simulink model "Vaxelriktare_Transducers"  (R2020b)
settings: Solver=VariableStepAuto  StartTime=0.0  StopTime=0.01  RelTol=1e-3
libraries: fl_lib x80, nesl_utility x32, ee_lib x3, SignalEditorBlockLib x1
(part 1 of 2)
settings Model: Creator=jenel  LastModifiedBy=jenel

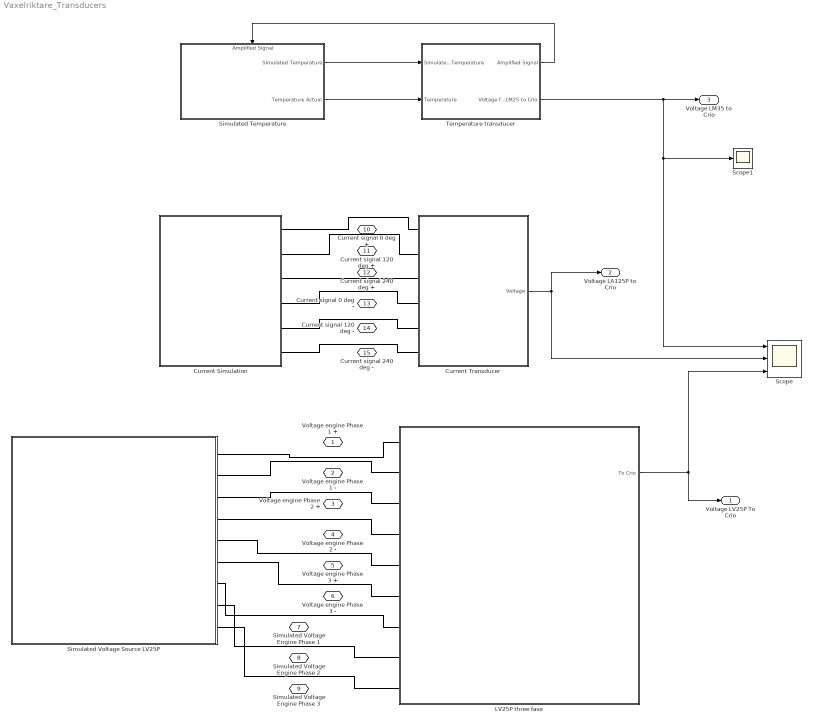
== system Vaxelriktare_Transducers ==
  Current Simulation : Subsystem
  Current Transducer : Subsystem
  LV25P three fase : Subsystem
  Scope : Scope  NumInputPorts=3
  Scope1 : Scope
  Simulated Temperature : Subsystem
      settings: PortSchema="{\"entries\":[{\"content\":{\"sides\":[{\"content\":{\"connectorIds\":[]},\"type\":\"ConnectorPlacement.EquallySpacedRectSide\",\"uuid\":\"52a7c08e-3c3e-468d-9a48-5db7e5268e65\"},{\"content\":{\"connectorIds\":[\"Out1\",\"Out2\"],\"side\":\"RIGHT\"},\"type\":\"ConnectorPlacement.EquallySpacedRectSide\",\"uuid\":\"cc00ce28-dfa9-4e8d-849b-21a8aa2e88a1\"},{\"content\":{\"connectorIds\":[\"In1\"],\"side\":\"TOP\"},\"type\":\"ConnectorPlacement.EquallySpacedRectSide\",\"uuid\":\"9c60ff72-e0ca-4689-b1b7-e246b8e0f47f\"},{\"content\":{\"connectorIds\":[],\"side\":\"HIDDEN\"},\"type\":\"ConnectorPlacement.EquallySpacedRectSide\",\"uuid\":\"4ba62725-7915-4645-8693-141a674fd740\"}]},\"type\":\"ConnectorPlacement.EquallySpacedConnector\",\"uuid\":\"cdec1a03-c0d5-4421-a983-90e94124080d\"}],\"packageUris\":[\"http://schema.mathworks.com/mf0/Connector/R2020b\"],\"version\":\"1.0\"}"
  Simulated Voltage Source LV25P : Subsystem
  Temperature transducer : Subsystem
  Voltage engine Phase 1 + : PMIOPort  Side=Right
  Voltage engine Phase 1 - : PMIOPort  Port=2  Side=Right
  Voltage engine Phase 2 + : PMIOPort  Port=3  Side=Right
  Voltage engine Phase 2 - : PMIOPort  Port=4  Side=Right
  Voltage engine Phase 3 + : PMIOPort  Port=5  Side=Right
  Voltage engine Phase 3 - : PMIOPort  Port=6  Side=Right
  Simulated Voltage Engine Phase 1 : PMIOPort  Port=7  Side=Right
  Simulated Voltage Engine Phase 2 : PMIOPort  Port=8  Side=Right
  Simulated Voltage Engine Phase 3 : PMIOPort  Port=9  Side=Right
  Current signal 0 deg + : PMIOPort  Port=10  Side=Right
  Current signal 120 deg + : PMIOPort  Port=11  Side=Right
  Current signal 240 deg + : PMIOPort  Port=12  Side=Right
  Current signal 0 deg - : PMIOPort  Port=13  Side=Right
  Current signal 120 deg - : PMIOPort  Port=14  Side=Right
  Current signal 240 deg - : PMIOPort  Port=15  Side=Right
  Voltage LV25P To Crio : Outport
  Voltage LA125P to Crio : Outport  Port=2
  Voltage LM35 to Crio : Outport  Port=3
  wires:
  LV25P three fase/1(To Crio) -> Voltage LV25P To Crio/1, Scope/3
  Current Transducer/1(Voltage) -> Scope/2, Voltage LA125P to Crio/1
  Simulated Temperature/1(Simulated Temperature) -> Temperature transducer/1(Simulated Temperature)
  Simulated Temperature/2(Temperature Actual) -> Temperature transducer/2(Temperature)
  Temperature transducer/1(Amplified Signal) -> Simulated Temperature/1(Amplified Signal)
  Temperature transducer/2(Voltage from LM25 to Crio) -> Voltage LM35 to Crio/1, Scope1/1, Scope/1
  connections:
  Simulated Voltage Source LV25P/RConn2 -- LV25P three fase/LConn2
  Simulated Voltage Source LV25P/RConn5 -- LV25P three fase/LConn5
  Simulated Voltage Source LV25P/RConn4 -- LV25P three fase/LConn4
  LV25P three fase/LConn6 -- Simulated Voltage Source LV25P/RConn6
  LV25P three fase/LConn7 -- Simulated Voltage Source LV25P/RConn7
  Simulated Voltage Source LV25P/RConn8 -- LV25P three fase/LConn8
  LV25P three fase/LConn3 -- Simulated Voltage Source LV25P/RConn3
  Simulated Voltage Source LV25P/RConn9 -- LV25P three fase/LConn9
  LV25P three fase/LConn1 -- Simulated Voltage Source LV25P/RConn1
  Current Simulation/LConn3 -- Current Transducer/LConn3
  Current Simulation/LConn2 -- Current Transducer/LConn2
  Current Simulation/LConn1 -- Current Transducer/LConn1
  Current Simulation/LConn6 -- Current Transducer/LConn6
  Current Simulation/LConn5 -- Current Transducer/LConn5
  Current Simulation/LConn4 -- Current Transducer/LConn4

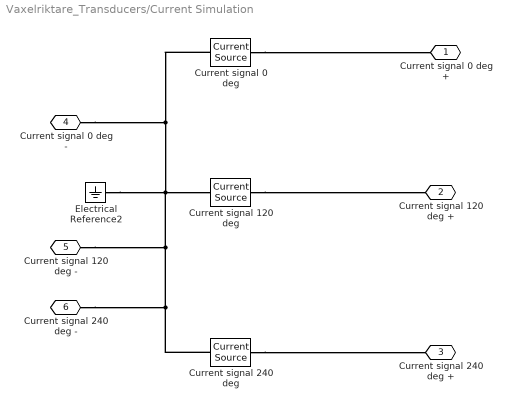
== system Vaxelriktare_Transducers/Current Simulation ==
  Current signal 0 deg : ee_lib/Sources/Current Source  dc_current=0 A  ac_current=200 mA  ac_shift=0 deg  ac_frequency=1000 Hz  noise_mode=0  PSD=0 A^2/Hz  repeatability=1  auto_seed=1274213173  user_seed=0  sample_time=1e-3 s  i_specify=off  i_priority=None  i=0 A  i_nominal_specify=off  i_nominal_unit=A  i_nominal_value=1  v_specify=off  v_priority=None  v=0 V  v_nominal_specify=off  v_nominal_unit=V  v_nominal_value=1
      settings: SourceProductBaseCode=PS
  Current signal 120 deg : ee_lib/Sources/Current Source  dc_current=0 A  ac_current=200 mA  ac_shift=120 deg  ac_frequency=1000 Hz  noise_mode=0  PSD=0 A^2/Hz  repeatability=1  auto_seed=1369142382  user_seed=0  sample_time=1e-3 s  i_specify=off  i_priority=None  i=0 A  i_nominal_specify=off  i_nominal_unit=A  i_nominal_value=1  v_specify=off  v_priority=None  v=0 V  v_nominal_specify=off  v_nominal_unit=V  v_nominal_value=1
      settings: SourceProductBaseCode=PS
  Current signal 240 deg : ee_lib/Sources/Current Source  dc_current=0 A  ac_current=200 mA  ac_shift=240 deg  ac_frequency=1000 Hz  noise_mode=0  PSD=0 A^2/Hz  repeatability=1  auto_seed=1821782361  user_seed=0  sample_time=1e-3 s  i_specify=off  i_priority=None  i=0 A  i_nominal_specify=off  i_nominal_unit=A  i_nominal_value=1  v_specify=off  v_priority=None  v=0 V  v_nominal_specify=off  v_nominal_unit=V  v_nominal_value=1
      settings: SourceProductBaseCode=PS
  Electrical Reference2 : fl_lib/Electrical/Electrical Elements/Electrical Reference
  Current signal 0 deg + : PMIOPort  Side=Left
  Current signal 120 deg + : PMIOPort  Port=2  Side=Left
  Current signal 240 deg + : PMIOPort  Port=3  Side=Left
  Current signal 0 deg - : PMIOPort  Port=4  Side=Left
  Current signal 120 deg - : PMIOPort  Port=5  Side=Left
  Current signal 240 deg - : PMIOPort  Port=6  Side=Left
  connections:
  Electrical Reference2/LConn1 -- Current signal 0 deg/RConn1 -- Current signal 0 deg -/RConn1 -- Current signal 240 deg/RConn1 -- Current signal 240 deg -/RConn1 -- Current signal 120 deg -/RConn1 -- Current signal 120 deg/RConn1
  Current signal 240 deg/LConn1 -- Current signal 240 deg +/RConn1
  Current signal 0 deg/LConn1 -- Current signal 0 deg +/RConn1
  Current signal 120 deg/LConn1 -- Current signal 120 deg +/RConn1

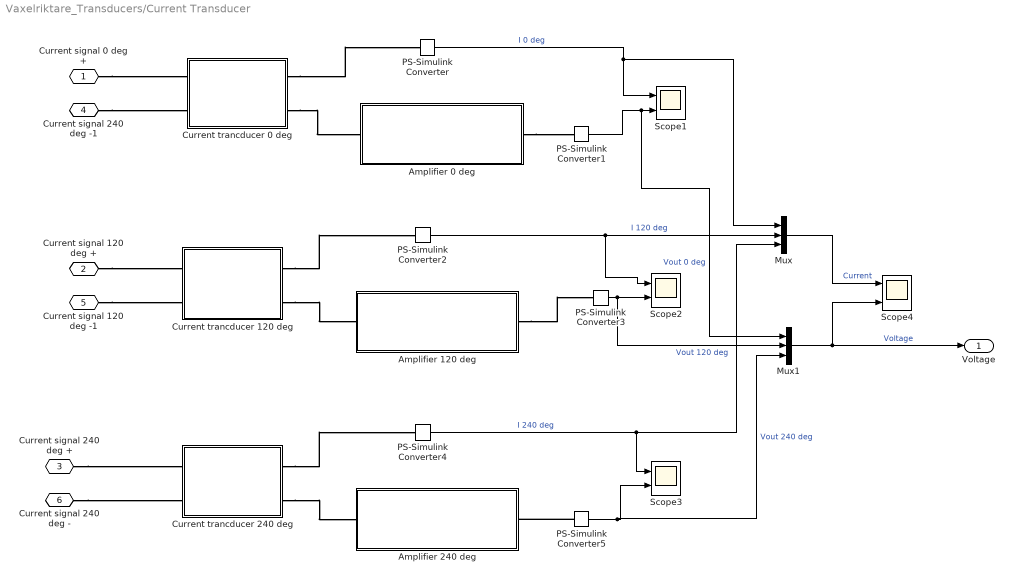
== system Vaxelriktare_Transducers/Current Transducer ==
  Amplifier 0 deg : Subsystem
  Amplifier 120 deg : Subsystem
  Amplifier 240 deg : Subsystem
  Current trancducer 0 deg : Subsystem
  Current trancducer 120 deg : Subsystem
  Current trancducer 240 deg : Subsystem
  Mux : Mux  Inputs=3
  Mux1 : Mux  Inputs=3
  PS-Simulink Converter{,1..5} (6 alike) : nesl_utility/PS-Simulink Converter  PhysicalDomain=network_engine_domain  SubClassName=ps_output  LeftPortType=input  RightPortType=output  PseudoPeriodic=off  Frequencies=[]  Unit=inherit  AffineConversion=off
  Scope{1..4} (4 alike) : Scope  NumInputPorts=2
  Current signal 0 deg + : PMIOPort  Side=Left
  Current signal 120 deg + : PMIOPort  Port=2  Side=Left
  Current signal 240 deg + : PMIOPort  Port=3  Side=Left
  Current signal 240 deg -1 : PMIOPort  Port=4  Side=Left
  Current signal 120 deg -1 : PMIOPort  Port=5  Side=Left
  Current signal 240 deg - : PMIOPort  Port=6  Side=Left
  Voltage : Outport
  wires:
  PS-Simulink Converter1/1 -> Mux1/1, Scope1/2  "Vout 0 deg"
  PS-Simulink Converter5/1 -> Mux1/3, Scope3/2  "Vout 240 deg"
  PS-Simulink Converter3/1 -> Mux1/2, Scope2/2  "Vout 120 deg"
  PS-Simulink Converter/1 -> Mux/1, Scope1/1  "I 0 deg"
  PS-Simulink Converter2/1 -> Scope2/1, Mux/2  "I 120 deg"
  PS-Simulink Converter4/1 -> Mux/3, Scope3/1  "I 240 deg"
  Mux1/1 -> Voltage/1, Scope4/2  "Voltage"
  Mux/1 -> Scope4/1  "Current"
  connections:
  Amplifier 120 deg/RConn1 -- PS-Simulink Converter3/LConn1
  Current trancducer 120 deg/RConn2 -- Amplifier 120 deg/LConn1
  Current trancducer 0 deg/RConn2 -- Amplifier 0 deg/LConn1
  Current trancducer 120 deg/RConn1 -- PS-Simulink Converter2/LConn1
  Current trancducer 0 deg/RConn1 -- PS-Simulink Converter/LConn1
  Current trancducer 240 deg/RConn2 -- Amplifier 240 deg/LConn1
  PS-Simulink Converter5/LConn1 -- Amplifier 240 deg/RConn1
  Amplifier 0 deg/RConn1 -- PS-Simulink Converter1/LConn1
  Current trancducer 240 deg/RConn1 -- PS-Simulink Converter4/LConn1
  Current signal 0 deg +/RConn1 -- Current trancducer 0 deg/LConn1
  Current signal 120 deg +/RConn1 -- Current trancducer 120 deg/LConn1
  Current signal 240 deg +/RConn1 -- Current trancducer 240 deg/LConn1
  Current signal 240 deg -/RConn1 -- Current trancducer 240 deg/LConn2
  Current signal 120 deg -1/RConn1 -- Current trancducer 120 deg/LConn2
  Current signal 240 deg -1/RConn1 -- Current trancducer 0 deg/LConn2

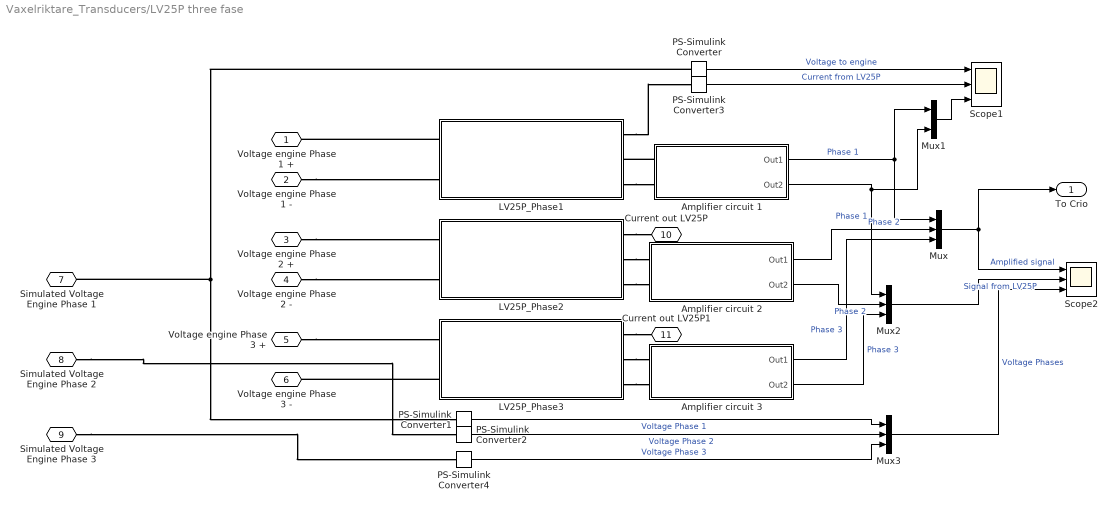
== system Vaxelriktare_Transducers/LV25P three fase ==
  Amplifier circuit 1 : Subsystem
  Amplifier circuit 2 : Subsystem
  Amplifier circuit 3 : Subsystem
  LV25P_Phase1 : Subsystem
  LV25P_Phase2 : Subsystem
  LV25P_Phase3 : Subsystem
  Mux : Mux  Inputs=3
  Mux1 : Mux  Inputs=2
  Mux2 : Mux  Inputs=3
  Mux3 : Mux  Inputs=3
  PS-Simulink Converter{,1..4} (5 alike) : nesl_utility/PS-Simulink Converter  PhysicalDomain=network_engine_domain  SubClassName=ps_output  LeftPortType=input  RightPortType=output  PseudoPeriodic=off  Frequencies=[]  Unit=inherit  AffineConversion=off
  Scope1 : Scope  NumInputPorts=3
  Scope2 : Scope  NumInputPorts=3
  Voltage engine Phase 1 + : PMIOPort  Side=Left
  Voltage engine Phase 1 - : PMIOPort  Port=2  Side=Left
  Voltage engine Phase 2 + : PMIOPort  Port=3  Side=Left
  Voltage engine Phase 2 - : PMIOPort  Port=4  Side=Left
  Voltage engine Phase 3 + : PMIOPort  Port=5  Side=Left
  Voltage engine Phase 3 - : PMIOPort  Port=6  Side=Left
  Simulated Voltage Engine Phase 1 : PMIOPort  Port=7  Side=Left
  Simulated Voltage Engine Phase 2 : PMIOPort  Port=8  Side=Left
  Simulated Voltage Engine Phase 3 : PMIOPort  Port=9  Side=Left
  Current out LV25P : PMIOPort  Port=10  Side=Right
  Current out LV25P1 : PMIOPort  Port=11  Side=Right
  To Crio : Outport
  wires:
  Mux3/1 -> Scope2/3  "Voltage Phases"
  PS-Simulink Converter1/1 -> Mux3/1  "Voltage Phase 1"
  Amplifier circuit 3/1(Out1) -> Mux/3  "Phase 3"
  Mux/1 -> To Crio/1, Scope2/1  "Amplified signal"
  PS-Simulink Converter4/1 -> Mux3/3  "Voltage Phase 3"
  Mux1/1 -> Scope1/3
  Amplifier circuit 1/2(Out2) -> Mux2/1, Mux1/2  "Phase 1"
  Amplifier circuit 2/2(Out2) -> Mux2/2  "Phase 2"
  PS-Simulink Converter2/1 -> Mux3/2  "Voltage Phase 2"
  PS-Simulink Converter/1 -> Scope1/1  "Voltage to engine"
  PS-Simulink Converter3/1 -> Scope1/2  "Current from LV25P"
  Amplifier circuit 2/1(Out1) -> Mux/2  "Phase 2"
  Amplifier circuit 3/2(Out2) -> Mux2/3  "Phase 3"
  Mux2/1 -> Scope2/2  "Signal from LV25P"
  Amplifier circuit 1/1(Out1) -> Mux1/1, Mux/1  "Phase 1"
  connections:
  Amplifier circuit 1/LConn1 -- LV25P_Phase1/RConn2
  Voltage engine Phase 2 -/RConn1 -- LV25P_Phase2/LConn2
  LV25P_Phase3/LConn2 -- Voltage engine Phase 3 -/RConn1
  LV25P_Phase2/RConn2 -- Amplifier circuit 2/LConn1
  PS-Simulink Converter/LConn1 -- PS-Simulink Converter1/LConn1 -- Simulated Voltage Engine Phase 1/RConn1
  LV25P_Phase1/RConn3 -- Amplifier circuit 1/LConn2
  LV25P_Phase2/RConn3 -- Amplifier circuit 2/LConn2
  Voltage engine Phase 3 +/RConn1 -- LV25P_Phase3/LConn1
  Simulated Voltage Engine Phase 3/RConn1 -- PS-Simulink Converter4/LConn1
  LV25P_Phase1/RConn1 -- PS-Simulink Converter3/LConn1
  Simulated Voltage Engine Phase 2/RConn1 -- PS-Simulink Converter2/LConn1
  Voltage engine Phase 2 +/RConn1 -- LV25P_Phase2/LConn1
  Voltage engine Phase 1 -/RConn1 -- LV25P_Phase1/LConn2
  LV25P_Phase1/LConn1 -- Voltage engine Phase 1 +/RConn1
  LV25P_Phase3/RConn2 -- Amplifier circuit 3/LConn1
  LV25P_Phase3/RConn3 -- Amplifier circuit 3/LConn2
  LV25P_Phase2/RConn1 -- Current out LV25P/RConn1
  LV25P_Phase3/RConn1 -- Current out LV25P1/RConn1

== system Vaxelriktare_Transducers/Simulated Temperature ==
  Amplified Signal : Inport
  Calculation temperature : Subsystem
  Mux1 : Mux  Inputs=2
  Temperature Simulation 2-150C : Subsystem
  Simulated Temperature : Outport
  Temperature Actual : Outport  Port=2
  wires:
  Temperature Simulation 2-150C/1(output) -> Temperature Actual/1, Mux1/2  "Temperature Actual"
  Calculation temperature/1(Temperature Measured) -> Mux1/1
  Mux1/1 -> Simulated Temperature/1
  Amplified Signal/1 -> Calculation temperature/1(Amplified Signal)

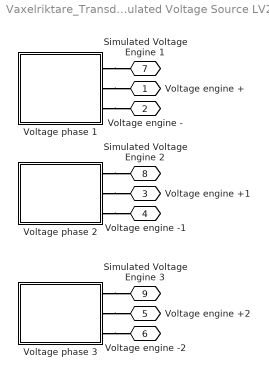
== system Vaxelriktare_Transducers/Simulated Voltage Source LV25P ==
  Voltage phase 1 : Subsystem
  Voltage phase 2 : Subsystem
  Voltage phase 3 : Subsystem
  Voltage engine + : PMIOPort  Side=Right
  Voltage engine - : PMIOPort  Port=2  Side=Right
  Voltage engine +1 : PMIOPort  Port=3  Side=Right
  Voltage engine -1 : PMIOPort  Port=4  Side=Right
  Voltage engine +2 : PMIOPort  Port=5  Side=Right
  Voltage engine -2 : PMIOPort  Port=6  Side=Right
  Simulated Voltage Engine 1 : PMIOPort  Port=7  Side=Right
  Simulated Voltage Engine 2 : PMIOPort  Port=8  Side=Right
  Simulated Voltage Engine 3 : PMIOPort  Port=9  Side=Right
  connections:
  Voltage phase 1/RConn3 -- Voltage engine -/RConn1
  Voltage phase 2/RConn3 -- Voltage engine -1/RConn1
  Voltage phase 2/RConn1 -- Simulated Voltage Engine 2/RConn1
  Voltage phase 3/RConn1 -- Simulated Voltage Engine 3/RConn1
  Voltage phase 1/RConn1 -- Simulated Voltage Engine 1/RConn1
  Voltage phase 1/RConn2 -- Voltage engine +/RConn1
  Voltage phase 3/RConn3 -- Voltage engine -2/RConn1
  Voltage phase 3/RConn2 -- Voltage engine +2/RConn1
  Voltage phase 2/RConn2 -- Voltage engine +1/RConn1

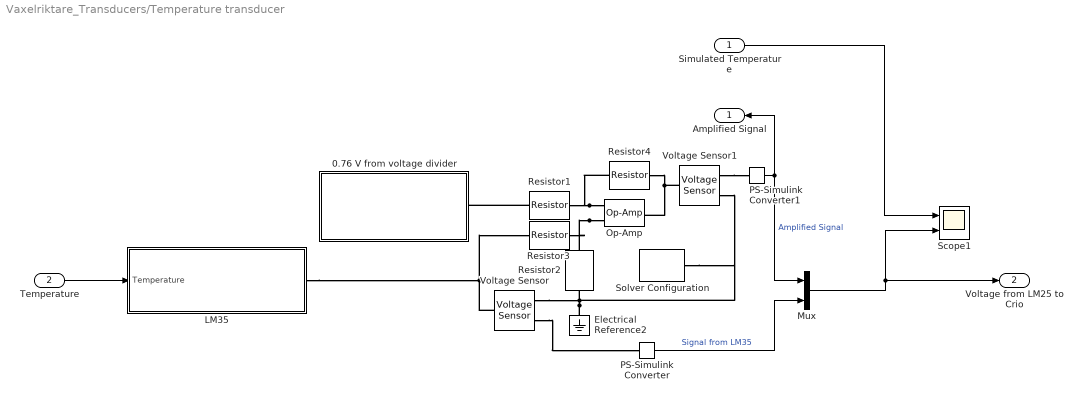
== system Vaxelriktare_Transducers/Temperature transducer ==
  Simulated Temperature : Inport
  Temperature : Inport  Port=2
  0.76 V from voltage divider : Subsystem
      settings: PortSchema="{\"entries\":[{\"content\":{\"sides\":[{\"content\":{\"connectorIds\":[]},\"type\":\"ConnectorPlacement.EquallySpacedRectSide\",\"uuid\":\"e1fed669-8d8a-41ed-8af4-1f1a704497c4\"},{\"content\":{\"connectorIds\":[],\"side\":\"RIGHT\"},\"type\":\"ConnectorPlacement.EquallySpacedRectSide\",\"uuid\":\"b0ee4a10-4969-4a29-9254-be0943d7fc2a\"},{\"content\":{\"connectorIds\":[],\"side\":\"TOP\"},\"type\":\"ConnectorPlacement.EquallySpacedRectSide\",\"uuid\":\"ce25e029-180c-4f91-8d66-56c124f96642\"},{\"content\":{\"connectorIds\":[\"RConn1\"],\"side\":\"BOTTOM\"},\"type\":\"ConnectorPlacement.EquallySpacedRectSide\",\"uuid\":\"d681aae5-3058-4c4e-809e-9c18db97e842\"},{\"content\":{\"connectorIds\":[],\"side\":\"HIDDEN\"},\"type\":\"ConnectorPlacement.EquallySpacedRectSide\",\"uuid\":\"286988fa-11ca-40d3-a957-1466b0eff549\"}]},\"type\":\"ConnectorPlacement.EquallySpacedConnector\",\"uuid\":\"e1bff037-5125-4ee2-a69f-b4bae47458cb\"}],\"packageUris\":[\"http://schema.mathworks.com/mf0/Connector/R2020b\"],\"version\":\"1.0\"}"
  Electrical Reference2 : fl_lib/Electrical/Electrical Elements/Electrical Reference
  LM35 : Subsystem
  Mux : Mux  Inputs=2
  Op-Amp : fl_lib/Electrical/Electrical Elements/Op-Amp  outI_specify=off  outI_priority=None  outI=0 A  outI_nominal_specify=off  outI_nominal_unit=A  outI_nominal_value=1
  PS-Simulink Converter : nesl_utility/PS-Simulink Converter  PhysicalDomain=network_engine_domain  SubClassName=ps_output  LeftPortType=input  RightPortType=output  PseudoPeriodic=off  Frequencies=[]  Unit=inherit  AffineConversion=off
  PS-Simulink Converter1 : nesl_utility/PS-Simulink Converter  PhysicalDomain=network_engine_domain  SubClassName=ps_output  LeftPortType=input  RightPortType=output  PseudoPeriodic=off  Frequencies=[]  Unit=inherit  AffineConversion=off
  Resistor1 : fl_lib/Electrical/Electrical Elements/Resistor  R=75 kOhm  i_specify=off  i_priority=None  i=0 A  i_nominal_specify=off  i_nominal_unit=A  i_nominal_value=1  v_specify=off  v_priority=None  v=0 V  v_nominal_specify=off  v_nominal_unit=V  v_nominal_value=1
  Resistor2 : fl_lib/Electrical/Electrical Elements/Resistor  R=1 MOhm  i_specify=off  i_priority=None  i=0 A  i_nominal_specify=off  i_nominal_unit=A  i_nominal_value=1  v_specify=off  v_priority=None  v=0 V  v_nominal_specify=off  v_nominal_unit=V  v_nominal_value=1
  Resistor3 : fl_lib/Electrical/Electrical Elements/Resistor  R=75 kOhm  i_specify=off  i_priority=None  i=0 A  i_nominal_specify=off  i_nominal_unit=A  i_nominal_value=1  v_specify=off  v_priority=None  v=0 V  v_nominal_specify=off  v_nominal_unit=V  v_nominal_value=1
  Resistor4 : fl_lib/Electrical/Electrical Elements/Resistor  R=1 MOhm  i_specify=off  i_priority=None  i=0 A  i_nominal_specify=off  i_nominal_unit=A  i_nominal_value=1  v_specify=off  v_priority=None  v=0 V  v_nominal_specify=off  v_nominal_unit=V  v_nominal_value=1
  Scope1 : Scope  NumInputPorts=2
  Solver Configuration : nesl_utility/Solver Configuration  PhysicalDomain=network_engine_domain  SubClassName=solver  LeftPortType=input  RightPortType=generic  Tones=[]  Harmonics=[]  SimulateNoise=off  Profile=off  UseLocalSampling=off  EnableSwitchedLinearOptims=on  FrequencyDomain=off  UseCCode=off  RelTol=0.001  AbsTol=1e-06  MinStep=1e-09  ToWorkspace=off  RevertToSquareIcSolve=off  NumHomotopyIterations=100  PhasorMode=off  PhasorModeNumHarmonics=1  DoDC=off  ResidualTolerance=1e-09  UseLocalSolver=off  LocalSolverChoice=NE_BACKWARD_EULER_ADVANCER  LocalSolverSampleTime=0.001  DoFixedCost=off  MaxNonlinIter=3  MaxModeIter=2  ComputeImpulses=off  ImpulseIterations=2  LinearAlgebra=auto  EquationFormulation=NE_TIME_EF  DelaysMemoryBudget=1024  AutomaticFiltering=on  FilteringTimeConstant=0.001  PartitionStorageMethod=AS_NEEDED  PartitionMemoryBudget=1024  PartitionMethod=ROBUST
  Voltage Sensor : fl_lib/Electrical/Electrical Sensors/Voltage Sensor
  Voltage Sensor1 : fl_lib/Electrical/Electrical Sensors/Voltage Sensor
  Amplified Signal : Outport
  Voltage from LM25 to Crio : Outport  Port=2
  wires:
  PS-Simulink Converter1/1 -> Amplified Signal/1, Mux/1  "Amplified Signal"
  Mux/1 -> Voltage from LM25 to Crio/1, Scope1/2
  Temperature/1 -> LM35/1(Temperature)
  PS-Simulink Converter/1 -> Mux/2  "Signal from LM35"
  Simulated Temperature/1 -> Scope1/1
  connections:
  Resistor2/RConn1 -- Voltage Sensor/RConn2 -- Solver Configuration/RConn1 -- Voltage Sensor1/RConn2 -- Electrical Reference2/LConn1
  Voltage Sensor/RConn1 -- PS-Simulink Converter/LConn1
  Voltage Sensor1/LConn1 -- Op-Amp/RConn1 -- Resistor4/LConn1
  Op-Amp/LConn1 -- Resistor1/LConn1 -- Resistor4/RConn1
  Op-Amp/LConn2 -- Resistor2/LConn1 -- Resistor3/LConn1
  LM35/RConn1 -- Resistor3/RConn1 -- Voltage Sensor/LConn1
  Resistor1/RConn1 -- 0.76 V from voltage divider/RConn1
  Voltage Sensor1/RConn1 -- PS-Simulink Converter1/LConn1

== system Vaxelriktare_Transducers/Current Transducer/Amplifier 0 deg ==
  Electrical Reference : fl_lib/Electrical/Electrical Elements/Electrical Reference
  Op-Amp : fl_lib/Electrical/Electrical Elements/Op-Amp  outI_specify=on  outI_priority=None  outI=0 A  outI_nominal_specify=off  outI_nominal_unit=A  outI_nominal_value=1
  R1 : fl_lib/Electrical/Electrical Elements/Resistor  R=1000 Ohm  i_specify=off  i_priority=None  i=0 A  i_nominal_specify=off  i_nominal_unit=A  i_nominal_value=1  v_specify=off  v_priority=None  v=0 V  v_nominal_specify=off  v_nominal_unit=V  v_nominal_value=1
  R2 : fl_lib/Electrical/Electrical Elements/Resistor  R=666.6667 Ohm  i_specify=off  i_priority=None  i=0 A  i_nominal_specify=off  i_nominal_unit=A  i_nominal_value=1  v_specify=off  v_priority=None  v=0 V  v_nominal_specify=off  v_nominal_unit=V  v_nominal_value=1
  Voltage Sensor : fl_lib/Electrical/Electrical Sensors/Voltage Sensor
  Vin : PMIOPort  Side=Left
  Vout : PMIOPort  Port=2  Side=Right
  connections:
  Op-Amp/RConn1 -- Voltage Sensor/LConn1 -- R2/RConn1
  Vin/RConn1 -- Op-Amp/LConn1
  Electrical Reference/LConn1 -- Voltage Sensor/RConn2 -- R1/RConn1
  R2/LConn1 -- R1/LConn1 -- Op-Amp/LConn2
  Voltage Sensor/RConn1 -- Vout/RConn1

== system Vaxelriktare_Transducers/Current Transducer/Amplifier 120 deg ==
  Electrical Reference : fl_lib/Electrical/Electrical Elements/Electrical Reference
  Op-Amp : fl_lib/Electrical/Electrical Elements/Op-Amp  outI_specify=on  outI_priority=None  outI=0 A  outI_nominal_specify=off  outI_nominal_unit=A  outI_nominal_value=1
  R1 : fl_lib/Electrical/Electrical Elements/Resistor  R=1000 Ohm  i_specify=off  i_priority=None  i=0 A  i_nominal_specify=off  i_nominal_unit=A  i_nominal_value=1  v_specify=off  v_priority=None  v=0 V  v_nominal_specify=off  v_nominal_unit=V  v_nominal_value=1
  R2 : fl_lib/Electrical/Electrical Elements/Resistor  R=666.6667 Ohm  i_specify=off  i_priority=None  i=0 A  i_nominal_specify=off  i_nominal_unit=A  i_nominal_value=1  v_specify=off  v_priority=None  v=0 V  v_nominal_specify=off  v_nominal_unit=V  v_nominal_value=1
  Voltage Sensor : fl_lib/Electrical/Electrical Sensors/Voltage Sensor
  Vin : PMIOPort  Side=Left
  Vout : PMIOPort  Port=2  Side=Right
  connections:
  Voltage Sensor/RConn1 -- Vout/RConn1
  Op-Amp/LConn2 -- R1/LConn1 -- R2/LConn1
  Voltage Sensor/RConn2 -- R1/RConn1 -- Electrical Reference/LConn1
  Vin/RConn1 -- Op-Amp/LConn1
  R2/RConn1 -- Voltage Sensor/LConn1 -- Op-Amp/RConn1

== system Vaxelriktare_Transducers/Current Transducer/Amplifier 240 deg ==
  Electrical Reference : fl_lib/Electrical/Electrical Elements/Electrical Reference
  Op-Amp : fl_lib/Electrical/Electrical Elements/Op-Amp  outI_specify=on  outI_priority=None  outI=0 A  outI_nominal_specify=off  outI_nominal_unit=A  outI_nominal_value=1
  R1 : fl_lib/Electrical/Electrical Elements/Resistor  R=1000 Ohm  i_specify=off  i_priority=None  i=0 A  i_nominal_specify=off  i_nominal_unit=A  i_nominal_value=1  v_specify=off  v_priority=None  v=0 V  v_nominal_specify=off  v_nominal_unit=V  v_nominal_value=1
  R2 : fl_lib/Electrical/Electrical Elements/Resistor  R=666.6667 Ohm  i_specify=off  i_priority=None  i=0 A  i_nominal_specify=off  i_nominal_unit=A  i_nominal_value=1  v_specify=off  v_priority=None  v=0 V  v_nominal_specify=off  v_nominal_unit=V  v_nominal_value=1
  Voltage Sensor : fl_lib/Electrical/Electrical Sensors/Voltage Sensor
  Vin : PMIOPort  Side=Left
  Vout : PMIOPort  Port=2  Side=Right
  connections:
  Op-Amp/RConn1 -- Voltage Sensor/LConn1 -- R2/RConn1
  Vin/RConn1 -- Op-Amp/LConn1
  Electrical Reference/LConn1 -- R1/RConn1 -- Voltage Sensor/RConn2
  R2/LConn1 -- R1/LConn1 -- Op-Amp/LConn2
  Voltage Sensor/RConn1 -- Vout/RConn1

== system Vaxelriktare_Transducers/Current Transducer/Current trancducer 0 deg ==
  Current Sensor : fl_lib/Electrical/Electrical Sensors/Current Sensor
  R3 : fl_lib/Electrical/Electrical Elements/Resistor  R=30 Ohm  i_specify=off  i_priority=None  i=0 A  i_nominal_specify=off  i_nominal_unit=A  i_nominal_value=1  v_specify=off  v_priority=None  v=0 V  v_nominal_specify=off  v_nominal_unit=V  v_nominal_value=1
  Current : PMIOPort  Side=Left
  Current Signal : PMIOPort  Port=2  Side=Right
  Vin : PMIOPort  Port=3  Side=Right
  Current signal 0 deg - : PMIOPort  Port=4  Side=Left
  connections:
  Current/RConn1 -- Current Sensor/LConn1
  Current Signal/RConn1 -- Current Sensor/RConn1
  Current Sensor/RConn2 -- Vin/RConn1 -- R3/LConn1
  R3/RConn1 -- Current signal 0 deg -/RConn1

== system Vaxelriktare_Transducers/Current Transducer/Current trancducer 120 deg ==
  Current Sensor : fl_lib/Electrical/Electrical Sensors/Current Sensor
  R3 : fl_lib/Electrical/Electrical Elements/Resistor  R=30 Ohm  i_specify=off  i_priority=None  i=0 A  i_nominal_specify=off  i_nominal_unit=A  i_nominal_value=1  v_specify=off  v_priority=None  v=0 V  v_nominal_specify=off  v_nominal_unit=V  v_nominal_value=1
  Solver Configuration : nesl_utility/Solver Configuration  PhysicalDomain=network_engine_domain  SubClassName=solver  LeftPortType=input  RightPortType=generic  Tones=[]  Harmonics=[]  SimulateNoise=off  Profile=off  UseLocalSampling=off  EnableSwitchedLinearOptims=on  FrequencyDomain=off  UseCCode=off  RelTol=0.001  AbsTol=1e-06  MinStep=1e-09  ToWorkspace=off  RevertToSquareIcSolve=off  NumHomotopyIterations=100  PhasorMode=off  PhasorModeNumHarmonics=1  DoDC=off  ResidualTolerance=1e-09  UseLocalSolver=off  LocalSolverChoice=NE_BACKWARD_EULER_ADVANCER  LocalSolverSampleTime=0.001  DoFixedCost=off  MaxNonlinIter=3  MaxModeIter=2  ComputeImpulses=off  ImpulseIterations=2  LinearAlgebra=auto  EquationFormulation=NE_TIME_EF  DelaysMemoryBudget=1024  AutomaticFiltering=on  FilteringTimeConstant=0.001  PartitionStorageMethod=AS_NEEDED  PartitionMemoryBudget=1024  PartitionMethod=ROBUST
  Current : PMIOPort  Side=Left
  Current signal 120 deg - : PMIOPort  Port=2  Side=Left
  Current Signal : PMIOPort  Port=3  Side=Right
  Vin : PMIOPort  Port=4  Side=Right
  connections:
  R3/RConn1 -- Current signal 120 deg -/RConn1 -- Solver Configuration/RConn1
  R3/LConn1 -- Vin/RConn1 -- Current Sensor/RConn2
  Current Signal/RConn1 -- Current Sensor/RConn1
  Current/RConn1 -- Current Sensor/LConn1

== system Vaxelriktare_Transducers/Current Transducer/Current trancducer 240 deg ==
  Current Sensor : fl_lib/Electrical/Electrical Sensors/Current Sensor
  R3 : fl_lib/Electrical/Electrical Elements/Resistor  R=30 Ohm  i_specify=off  i_priority=None  i=0 A  i_nominal_specify=off  i_nominal_unit=A  i_nominal_value=1  v_specify=off  v_priority=None  v=0 V  v_nominal_specify=off  v_nominal_unit=V  v_nominal_value=1
  Current : PMIOPort  Side=Left
  Current signal 240 deg - : PMIOPort  Port=2  Side=Left
  Current Signal : PMIOPort  Port=3  Side=Right
  Vin : PMIOPort  Port=4  Side=Right
  connections:
  Current/RConn1 -- Current Sensor/LConn1
  Current Signal/RConn1 -- Current Sensor/RConn1
  Current Sensor/RConn2 -- Vin/RConn1 -- R3/LConn1
  Current signal 240 deg -/RConn1 -- R3/RConn1

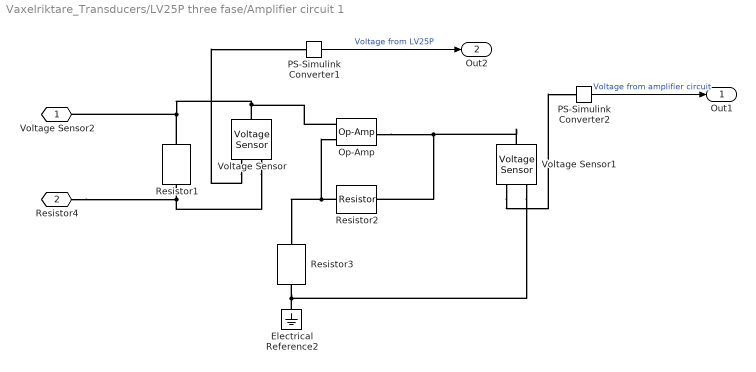
== system Vaxelriktare_Transducers/LV25P three fase/Amplifier circuit 1 ==
  Electrical Reference2 : fl_lib/Electrical/Electrical Elements/Electrical Reference
  Op-Amp : fl_lib/Electrical/Electrical Elements/Op-Amp  outI_specify=off  outI_priority=None  outI=0 A  outI_nominal_specify=off  outI_nominal_unit=A  outI_nominal_value=1
  PS-Simulink Converter1 : nesl_utility/PS-Simulink Converter  PhysicalDomain=network_engine_domain  SubClassName=ps_output  LeftPortType=input  RightPortType=output  PseudoPeriodic=off  Frequencies=[]  Unit=inherit  AffineConversion=off
  PS-Simulink Converter2 : nesl_utility/PS-Simulink Converter  PhysicalDomain=network_engine_domain  SubClassName=ps_output  LeftPortType=input  RightPortType=output  PseudoPeriodic=off  Frequencies=[]  Unit=inherit  AffineConversion=off
  Resistor1 : fl_lib/Electrical/Electrical Elements/Resistor  R=100 Ohm  i_specify=off  i_priority=None  i=0 A  i_nominal_specify=off  i_nominal_unit=A  i_nominal_value=1  v_specify=off  v_priority=None  v=0 V  v_nominal_specify=off  v_nominal_unit=V  v_nominal_value=1
  Resistor2 : fl_lib/Electrical/Electrical Elements/Resistor  R=30 kOhm  i_specify=off  i_priority=None  i=0 A  i_nominal_specify=off  i_nominal_unit=A  i_nominal_value=1  v_specify=off  v_priority=None  v=0 V  v_nominal_specify=off  v_nominal_unit=V  v_nominal_value=1
  Resistor3 : fl_lib/Electrical/Electrical Elements/Resistor  R=10 kOhm  i_specify=off  i_priority=None  i=0 A  i_nominal_specify=off  i_nominal_unit=A  i_nominal_value=1  v_specify=off  v_priority=None  v=0 V  v_nominal_specify=off  v_nominal_unit=V  v_nominal_value=1
  Voltage Sensor : fl_lib/Electrical/Electrical Sensors/Voltage Sensor
  Voltage Sensor1 : fl_lib/Electrical/Electrical Sensors/Voltage Sensor
  Voltage Sensor2 : PMIOPort  Side=Left
  Resistor4 : PMIOPort  Port=2  Side=Left
  Out1 : Outport
  Out2 : Outport  Port=2
  wires:
  PS-Simulink Converter2/1 -> Out1/1  "Voltage from amplifier circuit"
  PS-Simulink Converter1/1 -> Out2/1  "Voltage from LV25P"
  connections:
  Resistor1/LConn1 -- Op-Amp/LConn1 -- Voltage Sensor/LConn1 -- Voltage Sensor2/RConn1
  Op-Amp/RConn1 -- Voltage Sensor1/LConn1 -- Resistor2/RConn1
  Voltage Sensor/RConn2 -- Resistor4/RConn1 -- Resistor1/RConn1
  Voltage Sensor1/RConn1 -- PS-Simulink Converter2/LConn1
  Electrical Reference2/LConn1 -- Voltage Sensor1/RConn2 -- Resistor3/RConn1
  Resistor2/LConn1 -- Op-Amp/LConn2 -- Resistor3/LConn1
  Voltage Sensor/RConn1 -- PS-Simulink Converter1/LConn1

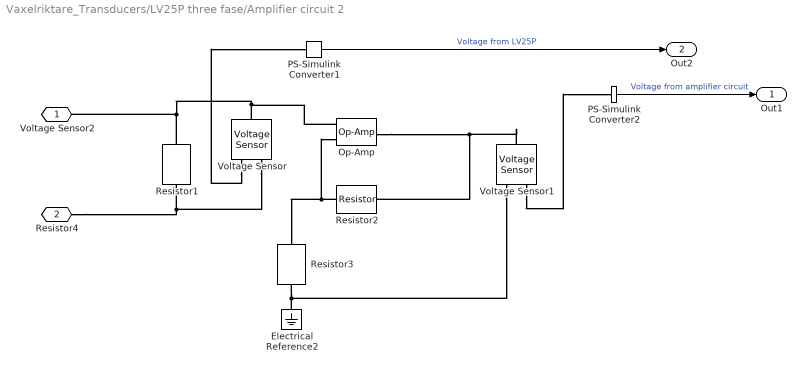
== system Vaxelriktare_Transducers/LV25P three fase/Amplifier circuit 2 ==
  Electrical Reference2 : fl_lib/Electrical/Electrical Elements/Electrical Reference
  Op-Amp : fl_lib/Electrical/Electrical Elements/Op-Amp  outI_specify=off  outI_priority=None  outI=0 A  outI_nominal_specify=off  outI_nominal_unit=A  outI_nominal_value=1
  PS-Simulink Converter1 : nesl_utility/PS-Simulink Converter  PhysicalDomain=network_engine_domain  SubClassName=ps_output  LeftPortType=input  RightPortType=output  PseudoPeriodic=off  Frequencies=[]  Unit=inherit  AffineConversion=off
  PS-Simulink Converter2 : nesl_utility/PS-Simulink Converter  PhysicalDomain=network_engine_domain  SubClassName=ps_output  LeftPortType=input  RightPortType=output  PseudoPeriodic=off  Frequencies=[]  Unit=inherit  AffineConversion=off
  Resistor1 : fl_lib/Electrical/Electrical Elements/Resistor  R=100 Ohm  i_specify=off  i_priority=None  i=0 A  i_nominal_specify=off  i_nominal_unit=A  i_nominal_value=1  v_specify=off  v_priority=None  v=0 V  v_nominal_specify=off  v_nominal_unit=V  v_nominal_value=1
  Resistor2 : fl_lib/Electrical/Electrical Elements/Resistor  R=30 kOhm  i_specify=off  i_priority=None  i=0 A  i_nominal_specify=off  i_nominal_unit=A  i_nominal_value=1  v_specify=off  v_priority=None  v=0 V  v_nominal_specify=off  v_nominal_unit=V  v_nominal_value=1
  Resistor3 : fl_lib/Electrical/Electrical Elements/Resistor  R=10 kOhm  i_specify=off  i_priority=None  i=0 A  i_nominal_specify=off  i_nominal_unit=A  i_nominal_value=1  v_specify=off  v_priority=None  v=0 V  v_nominal_specify=off  v_nominal_unit=V  v_nominal_value=1
  Voltage Sensor : fl_lib/Electrical/Electrical Sensors/Voltage Sensor
  Voltage Sensor1 : fl_lib/Electrical/Electrical Sensors/Voltage Sensor
  Voltage Sensor2 : PMIOPort  Side=Left
  Resistor4 : PMIOPort  Port=2  Side=Left
  Out1 : Outport
  Out2 : Outport  Port=2
  wires:
  PS-Simulink Converter2/1 -> Out1/1  "Voltage from amplifier circuit"
  PS-Simulink Converter1/1 -> Out2/1  "Voltage from LV25P"
  connections:
  Op-Amp/LConn1 -- Voltage Sensor/LConn1 -- Resistor1/LConn1 -- Voltage Sensor2/RConn1
  Op-Amp/RConn1 -- Voltage Sensor1/LConn1 -- Resistor2/RConn1
  Voltage Sensor/RConn2 -- Resistor1/RConn1 -- Resistor4/RConn1
  Voltage Sensor1/RConn1 -- PS-Simulink Converter2/LConn1
  Electrical Reference2/LConn1 -- Resistor3/RConn1 -- Voltage Sensor1/RConn2
  Resistor2/LConn1 -- Op-Amp/LConn2 -- Resistor3/LConn1
  Voltage Sensor/RConn1 -- PS-Simulink Converter1/LConn1

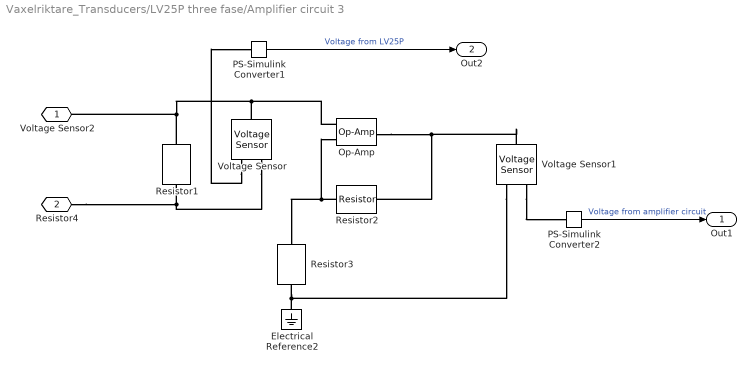
== system Vaxelriktare_Transducers/LV25P three fase/Amplifier circuit 3 ==
  Electrical Reference2 : fl_lib/Electrical/Electrical Elements/Electrical Reference
  Op-Amp : fl_lib/Electrical/Electrical Elements/Op-Amp  outI_specify=off  outI_priority=None  outI=0 A  outI_nominal_specify=off  outI_nominal_unit=A  outI_nominal_value=1
  PS-Simulink Converter1 : nesl_utility/PS-Simulink Converter  PhysicalDomain=network_engine_domain  SubClassName=ps_output  LeftPortType=input  RightPortType=output  PseudoPeriodic=off  Frequencies=[]  Unit=inherit  AffineConversion=off
  PS-Simulink Converter2 : nesl_utility/PS-Simulink Converter  PhysicalDomain=network_engine_domain  SubClassName=ps_output  LeftPortType=input  RightPortType=output  PseudoPeriodic=off  Frequencies=[]  Unit=inherit  AffineConversion=off
  Resistor1 : fl_lib/Electrical/Electrical Elements/Resistor  R=100 Ohm  i_specify=off  i_priority=None  i=0 A  i_nominal_specify=off  i_nominal_unit=A  i_nominal_value=1  v_specify=off  v_priority=None  v=0 V  v_nominal_specify=off  v_nominal_unit=V  v_nominal_value=1
  Resistor2 : fl_lib/Electrical/Electrical Elements/Resistor  R=30 kOhm  i_specify=off  i_priority=None  i=0 A  i_nominal_specify=off  i_nominal_unit=A  i_nominal_value=1  v_specify=off  v_priority=None  v=0 V  v_nominal_specify=off  v_nominal_unit=V  v_nominal_value=1
  Resistor3 : fl_lib/Electrical/Electrical Elements/Resistor  R=10 kOhm  i_specify=off  i_priority=None  i=0 A  i_nominal_specify=off  i_nominal_unit=A  i_nominal_value=1  v_specify=off  v_priority=None  v=0 V  v_nominal_specify=off  v_nominal_unit=V  v_nominal_value=1
  Voltage Sensor : fl_lib/Electrical/Electrical Sensors/Voltage Sensor
  Voltage Sensor1 : fl_lib/Electrical/Electrical Sensors/Voltage Sensor
  Voltage Sensor2 : PMIOPort  Side=Left
  Resistor4 : PMIOPort  Port=2  Side=Left
  Out1 : Outport
  Out2 : Outport  Port=2
  wires:
  PS-Simulink Converter2/1 -> Out1/1  "Voltage from amplifier circuit"
  PS-Simulink Converter1/1 -> Out2/1  "Voltage from LV25P"
  connections:
  Op-Amp/LConn1 -- Voltage Sensor/LConn1 -- Resistor1/LConn1 -- Voltage Sensor2/RConn1
  Op-Amp/RConn1 -- Voltage Sensor1/LConn1 -- Resistor2/RConn1
  Voltage Sensor/RConn2 -- Resistor4/RConn1 -- Resistor1/RConn1
  Voltage Sensor1/RConn1 -- PS-Simulink Converter2/LConn1
  Electrical Reference2/LConn1 -- Voltage Sensor1/RConn2 -- Resistor3/RConn1
  Resistor2/LConn1 -- Op-Amp/LConn2 -- Resistor3/LConn1
  Voltage Sensor/RConn1 -- PS-Simulink Converter1/LConn1

== system Vaxelriktare_Transducers/LV25P three fase/LV25P_Phase1 ==
  Current Sensor1 : fl_lib/Electrical/Electrical Sensors/Current Sensor
  Electrical Reference1 : fl_lib/Electrical/Electrical Elements/Electrical Reference
  Voltage-Controlled Current Source : fl_lib/Electrical/Electrical Sources/Voltage-Controlled Current Source  K=0.000125 1/Ohm  v1_specify=off  v1_priority=None  v1=0 V  v1_nominal_specify=off  v1_nominal_unit=V  v1_nominal_value=1  i2_specify=off  i2_priority=None  i2=0 A  i2_nominal_specify=off  i2_nominal_unit=A  i2_nominal_value=1
      settings: SourceProductBaseCode=SS  InternalSimscapePortConfiguration="{\"Bottom\":[],\"Left\":[{\"id\":\"p1\",\"label\":\"+\",\"type\":\"foundation.electrical.electrical\"},{\"id\":\"head\",\"label\":\"\",\"type\":\"foundation.electrical.electrical\"}],\"Right\":[{\"id\":\"n1\",\"label\":\"-\",\"type\":\"foundation.electrical.electrical\"},{\"id\":\"tail\",\"label\":\"\",\"type\":\"foundation.electrical.electrical\"}],\"Top\":[]}"
  Voltage engine + : PMIOPort  Side=Left
  Voltage engine - : PMIOPort  Port=2  Side=Left
  Current out LV25P : PMIOPort  Port=3  Side=Right
  Current + : PMIOPort  Port=4  Side=Right
  Current - : PMIOPort  Port=5  Side=Right
  connections:
  Current -/RConn1 -- Voltage-Controlled Current Source/RConn2 -- Electrical Reference1/LConn1
  Voltage-Controlled Current Source/LConn2 -- Current Sensor1/LConn1
  Current +/RConn1 -- Current Sensor1/RConn2
  Voltage-Controlled Current Source/RConn1 -- Voltage engine -/RConn1
  Current Sensor1/RConn1 -- Current out LV25P/RConn1
  Voltage-Controlled Current Source/LConn1 -- Voltage engine +/RConn1

== system Vaxelriktare_Transducers/LV25P three fase/LV25P_Phase2 ==
  Current Sensor1 : fl_lib/Electrical/Electrical Sensors/Current Sensor
  Electrical Reference1 : fl_lib/Electrical/Electrical Elements/Electrical Reference
  Voltage-Controlled Current Source : fl_lib/Electrical/Electrical Sources/Voltage-Controlled Current Source  K=0.000125 1/Ohm  v1_specify=off  v1_priority=None  v1=0 V  v1_nominal_specify=off  v1_nominal_unit=V  v1_nominal_value=1  i2_specify=off  i2_priority=None  i2=0 A  i2_nominal_specify=off  i2_nominal_unit=A  i2_nominal_value=1
      settings: SourceProductBaseCode=SS  InternalSimscapePortConfiguration="{\"Bottom\":[],\"Left\":[{\"id\":\"p1\",\"label\":\"+\",\"type\":\"foundation.electrical.electrical\"},{\"id\":\"head\",\"label\":\"\",\"type\":\"foundation.electrical.electrical\"}],\"Right\":[{\"id\":\"n1\",\"label\":\"-\",\"type\":\"foundation.electrical.electrical\"},{\"id\":\"tail\",\"label\":\"\",\"type\":\"foundation.electrical.electrical\"}],\"Top\":[]}"
  Voltage engine + : PMIOPort  Side=Left
  Voltage engine - : PMIOPort  Port=2  Side=Left
  Current out LV25P : PMIOPort  Port=3  Side=Right
  Current + : PMIOPort  Port=4  Side=Right
  Current - : PMIOPort  Port=5  Side=Right
  connections:
  Current -/RConn1 -- Electrical Reference1/LConn1 -- Voltage-Controlled Current Source/RConn2
  Voltage-Controlled Current Source/LConn2 -- Current Sensor1/LConn1
  Current +/RConn1 -- Current Sensor1/RConn2
  Voltage-Controlled Current Source/RConn1 -- Voltage engine -/RConn1
  Current Sensor1/RConn1 -- Current out LV25P/RConn1
  Voltage-Controlled Current Source/LConn1 -- Voltage engine +/RConn1

== system Vaxelriktare_Transducers/LV25P three fase/LV25P_Phase3 ==
  Current Sensor1 : fl_lib/Electrical/Electrical Sensors/Current Sensor
  Electrical Reference1 : fl_lib/Electrical/Electrical Elements/Electrical Reference
  Voltage-Controlled Current Source : fl_lib/Electrical/Electrical Sources/Voltage-Controlled Current Source  K=0.000125 1/Ohm  v1_specify=off  v1_priority=None  v1=0 V  v1_nominal_specify=off  v1_nominal_unit=V  v1_nominal_value=1  i2_specify=off  i2_priority=None  i2=0 A  i2_nominal_specify=off  i2_nominal_unit=A  i2_nominal_value=1
      settings: SourceProductBaseCode=SS  InternalSimscapePortConfiguration="{\"Bottom\":[],\"Left\":[{\"id\":\"p1\",\"label\":\"+\",\"type\":\"foundation.electrical.electrical\"},{\"id\":\"head\",\"label\":\"\",\"type\":\"foundation.electrical.electrical\"}],\"Right\":[{\"id\":\"n1\",\"label\":\"-\",\"type\":\"foundation.electrical.electrical\"},{\"id\":\"tail\",\"label\":\"\",\"type\":\"foundation.electrical.electrical\"}],\"Top\":[]}"
  Voltage engine + : PMIOPort  Side=Left
  Voltage engine - : PMIOPort  Port=2  Side=Left
  Current out LV25P : PMIOPort  Port=3  Side=Right
  Current + : PMIOPort  Port=4  Side=Right
  Current - : PMIOPort  Port=5  Side=Right
  connections:
  Current -/RConn1 -- Electrical Reference1/LConn1 -- Voltage-Controlled Current Source/RConn2
  Voltage-Controlled Current Source/LConn2 -- Current Sensor1/LConn1
  Current +/RConn1 -- Current Sensor1/RConn2
  Voltage-Controlled Current Source/RConn1 -- Voltage engine -/RConn1
  Current Sensor1/RConn1 -- Current out LV25P/RConn1
  Voltage-Controlled Current Source/LConn1 -- Voltage engine +/RConn1

== system Vaxelriktare_Transducers/Simulated Temperature/Calculation temperature ==
  Amplified Signal : Inport
  Add : Sum
  Constant : Constant  Value=10
  Gain : Gain  Gain=7.5
  Temperature Measured : Outport
  wires:
  Constant/1 -> Add/2
  Add/1 -> Gain/1
  Gain/1 -> Temperature Measured/1  "Temperature Measured"
  Amplified Signal/1 -> Add/1

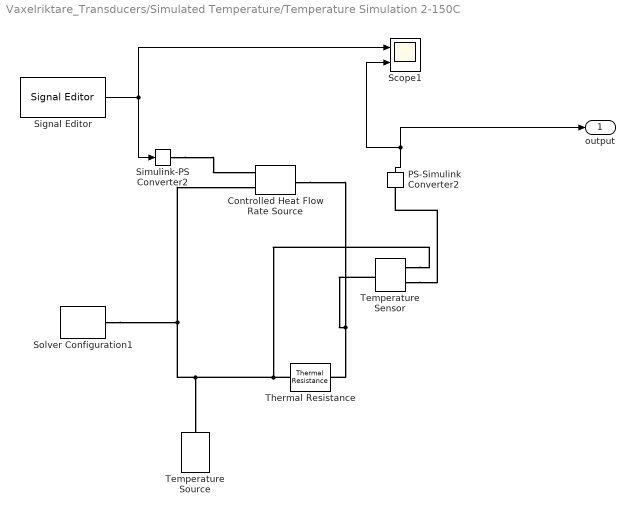
== system Vaxelriktare_Transducers/Simulated Temperature/Temperature Simulation 2-150C ==
  Controlled Heat Flow Rate Source : fl_lib/Thermal/Thermal Sources/Controlled Heat Flow Rate Source
  PS-Simulink Converter2 : nesl_utility/PS-Simulink Converter  PhysicalDomain=network_engine_domain  SubClassName=ps_output  LeftPortType=input  RightPortType=output  PseudoPeriodic=off  Frequencies=[]  Unit=inherit  AffineConversion=off
  Scope1 : Scope  NumInputPorts=2
  Signal Editor : SignalEditorBlockLib/Signal Editor  FileName=Temperature_Data.mat  ActiveScenario=Scenario  ActiveSignal=Signal 1  IsBus=off  OutputBusObjectStr=Bus: BusObject  SampleTime=0  ZeroCross=off  OutputAfterFinalValue=Setting to zero  Unit=inherit  PreserveSignalName=on
  Simulink-PS Converter2 : nesl_utility/Simulink-PS Converter  PhysicalDomain=network_engine_domain  SubClassName=ps_input  LeftPortType=input  RightPortType=output  PseudoPeriodic=off  Frequencies=[]  NoiseDistribution=none  NoiseParameters=[]  Unit=1  AffineConversion=off  FilteringAndDerivatives=provide  SimscapeFilterOrder=1  InputFilterTimeConstant=0.001  UdotUserProvided=0
  Solver Configuration1 : nesl_utility/Solver Configuration  PhysicalDomain=network_engine_domain  SubClassName=solver  LeftPortType=input  RightPortType=generic  Tones=[]  Harmonics=[]  SimulateNoise=off  Profile=off  UseLocalSampling=off  EnableSwitchedLinearOptims=on  FrequencyDomain=off  UseCCode=off  RelTol=0.001  AbsTol=1e-06  MinStep=1e-09  ToWorkspace=off  RevertToSquareIcSolve=off  NumHomotopyIterations=100  PhasorMode=off  PhasorModeNumHarmonics=1  DoDC=off  ResidualTolerance=1e-09  UseLocalSolver=off  LocalSolverChoice=NE_BACKWARD_EULER_ADVANCER  LocalSolverSampleTime=0.001  DoFixedCost=off  MaxNonlinIter=3  MaxModeIter=2  ComputeImpulses=off  ImpulseIterations=2  LinearAlgebra=auto  EquationFormulation=NE_TIME_EF  DelaysMemoryBudget=1024  AutomaticFiltering=on  FilteringTimeConstant=0.001  PartitionStorageMethod=AS_NEEDED  PartitionMemoryBudget=1024  PartitionMethod=ROBUST
  Temperature Sensor : fl_lib/Thermal/Thermal Sensors/Temperature Sensor
  Temperature Source : fl_lib/Thermal/Thermal Sources/Temperature Source  temperature=293.15 K
  Thermal Resistance : fl_lib/Thermal/Thermal Elements/Thermal Resistance  resistance=0.98 K/W  T_specify=off  T_priority=None  T=0 K  T_nominal_specify=off  T_nominal_unit=K  T_nominal_value=1  Q_specify=off  Q_priority=None  Q=0 W  Q_nominal_specify=off  Q_nominal_unit=W  Q_nominal_value=1
      settings: SourceProductBaseCode=SS
  output : Outport
  wires:
  PS-Simulink Converter2/1 -> output/1, Scope1/2
  Signal Editor/1 -> Simulink-PS Converter2/1, Scope1/1
  connections:
  Temperature Sensor/LConn1 -- Thermal Resistance/RConn1 -- Controlled Heat Flow Rate Source/LConn1
  Thermal Resistance/LConn1 -- Temperature Sensor/RConn1 -- Temperature Source/LConn1 -- Solver Configuration1/RConn1 -- Controlled Heat Flow Rate Source/RConn2
  Simulink-PS Converter2/RConn1 -- Controlled Heat Flow Rate Source/RConn1
  Temperature Sensor/RConn2 -- PS-Simulink Converter2/LConn1

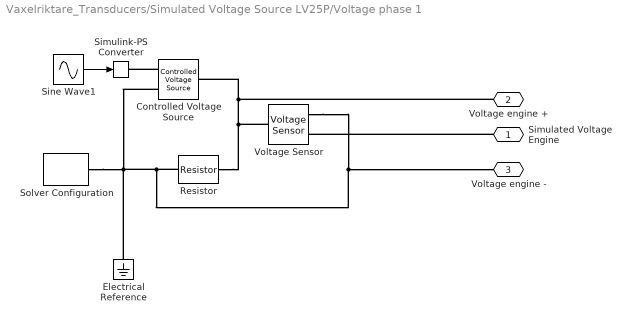
== system Vaxelriktare_Transducers/Simulated Voltage Source LV25P/Voltage phase 1 ==
  Controlled Voltage Source : fl_lib/Electrical/Electrical Sources/Controlled Voltage Source
  Electrical Reference : fl_lib/Electrical/Electrical Elements/Electrical Reference
  Resistor : fl_lib/Electrical/Electrical Elements/Resistor  R=10 Ohm  i_specify=off  i_priority=None  i=0 A  i_nominal_specify=off  i_nominal_unit=A  i_nominal_value=1  v_specify=off  v_priority=None  v=0 V  v_nominal_specify=off  v_nominal_unit=V  v_nominal_value=1
  Simulink-PS Converter : nesl_utility/Simulink-PS Converter  PhysicalDomain=network_engine_domain  SubClassName=ps_input  LeftPortType=input  RightPortType=output  PseudoPeriodic=off  Frequencies=[]  NoiseDistribution=none  NoiseParameters=[]  Unit=1  AffineConversion=off  FilteringAndDerivatives=provide  SimscapeFilterOrder=1  InputFilterTimeConstant=0.001  UdotUserProvided=0
  Sine Wave1 : Sin  Amplitude=200  Frequency=1000  SampleTime=0
  Solver Configuration : nesl_utility/Solver Configuration  PhysicalDomain=network_engine_domain  SubClassName=solver  LeftPortType=input  RightPortType=generic  Tones=[]  Harmonics=[]  SimulateNoise=off  Profile=off  UseLocalSampling=off  EnableSwitchedLinearOptims=on  FrequencyDomain=off  UseCCode=off  RelTol=0.001  AbsTol=1e-06  MinStep=1e-09  ToWorkspace=off  RevertToSquareIcSolve=off  NumHomotopyIterations=100  PhasorMode=off  PhasorModeNumHarmonics=1  DoDC=off  ResidualTolerance=1e-09  UseLocalSolver=off  LocalSolverChoice=NE_BACKWARD_EULER_ADVANCER  LocalSolverSampleTime=0.001  DoFixedCost=off  MaxNonlinIter=3  MaxModeIter=2  ComputeImpulses=off  ImpulseIterations=2  LinearAlgebra=auto  EquationFormulation=NE_TIME_EF  DelaysMemoryBudget=1024  AutomaticFiltering=on  FilteringTimeConstant=0.001  PartitionStorageMethod=AS_NEEDED  PartitionMemoryBudget=1024  PartitionMethod=ROBUST
  Voltage Sensor : fl_lib/Electrical/Electrical Sensors/Voltage Sensor
  Simulated Voltage Engine : PMIOPort  Side=Right
  Voltage engine + : PMIOPort  Port=2  Side=Right
  Voltage engine - : PMIOPort  Port=3  Side=Right
  wires:
  Sine Wave1/1 -> Simulink-PS Converter/1
  connections:
  Controlled Voltage Source/RConn1 -- Simulink-PS Converter/RConn1
  Simulated Voltage Engine/RConn1 -- Voltage Sensor/RConn1
  Voltage Sensor/LConn1 -- Controlled Voltage Source/LConn1 -- Voltage engine +/RConn1 -- Resistor/RConn1
  Resistor/LConn1 -- Voltage Sensor/RConn2 -- Voltage engine -/RConn1 -- Electrical Reference/LConn1 -- Solver Configuration/RConn1 -- Controlled Voltage Source/RConn2

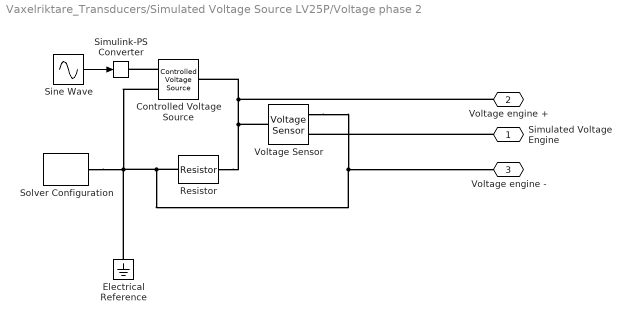
== system Vaxelriktare_Transducers/Simulated Voltage Source LV25P/Voltage phase 2 ==
  Controlled Voltage Source : fl_lib/Electrical/Electrical Sources/Controlled Voltage Source
  Electrical Reference : fl_lib/Electrical/Electrical Elements/Electrical Reference
  Resistor : fl_lib/Electrical/Electrical Elements/Resistor  R=10 Ohm  i_specify=off  i_priority=None  i=0 A  i_nominal_specify=off  i_nominal_unit=A  i_nominal_value=1  v_specify=off  v_priority=None  v=0 V  v_nominal_specify=off  v_nominal_unit=V  v_nominal_value=1
  Simulink-PS Converter : nesl_utility/Simulink-PS Converter  PhysicalDomain=network_engine_domain  SubClassName=ps_input  LeftPortType=input  RightPortType=output  PseudoPeriodic=off  Frequencies=[]  NoiseDistribution=none  NoiseParameters=[]  Unit=1  AffineConversion=off  FilteringAndDerivatives=provide  SimscapeFilterOrder=1  InputFilterTimeConstant=0.001  UdotUserProvided=0
  Sine Wave : Sin  Amplitude=200  Frequency=1000  Phase=2*pi/3  SampleTime=0
  Solver Configuration : nesl_utility/Solver Configuration  PhysicalDomain=network_engine_domain  SubClassName=solver  LeftPortType=input  RightPortType=generic  Tones=[]  Harmonics=[]  SimulateNoise=off  Profile=off  UseLocalSampling=off  EnableSwitchedLinearOptims=on  FrequencyDomain=off  UseCCode=off  RelTol=0.001  AbsTol=1e-06  MinStep=1e-09  ToWorkspace=off  RevertToSquareIcSolve=off  NumHomotopyIterations=100  PhasorMode=off  PhasorModeNumHarmonics=1  DoDC=off  ResidualTolerance=1e-09  UseLocalSolver=off  LocalSolverChoice=NE_BACKWARD_EULER_ADVANCER  LocalSolverSampleTime=0.001  DoFixedCost=off  MaxNonlinIter=3  MaxModeIter=2  ComputeImpulses=off  ImpulseIterations=2  LinearAlgebra=auto  EquationFormulation=NE_TIME_EF  DelaysMemoryBudget=1024  AutomaticFiltering=on  FilteringTimeConstant=0.001  PartitionStorageMethod=AS_NEEDED  PartitionMemoryBudget=1024  PartitionMethod=ROBUST
  Voltage Sensor : fl_lib/Electrical/Electrical Sensors/Voltage Sensor
  Simulated Voltage Engine : PMIOPort  Side=Right
  Voltage engine + : PMIOPort  Port=2  Side=Right
  Voltage engine - : PMIOPort  Port=3  Side=Right
  wires:
  Sine Wave/1 -> Simulink-PS Converter/1
  connections:
  Controlled Voltage Source/RConn1 -- Simulink-PS Converter/RConn1
  Simulated Voltage Engine/RConn1 -- Voltage Sensor/RConn1
  Resistor/RConn1 -- Voltage Sensor/LConn1 -- Voltage engine +/RConn1 -- Controlled Voltage Source/LConn1
  Electrical Reference/LConn1 -- Solver Configuration/RConn1 -- Controlled Voltage Source/RConn2 -- Resistor/LConn1 -- Voltage engine -/RConn1 -- Voltage Sensor/RConn2

== system Vaxelriktare_Transducers/Simulated Voltage Source LV25P/Voltage phase 3 ==
  Controlled Voltage Source : fl_lib/Electrical/Electrical Sources/Controlled Voltage Source
  Electrical Reference : fl_lib/Electrical/Electrical Elements/Electrical Reference
  Resistor : fl_lib/Electrical/Electrical Elements/Resistor  R=10 Ohm  i_specify=off  i_priority=None  i=0 A  i_nominal_specify=off  i_nominal_unit=A  i_nominal_value=1  v_specify=off  v_priority=None  v=0 V  v_nominal_specify=off  v_nominal_unit=V  v_nominal_value=1
  Simulink-PS Converter : nesl_utility/Simulink-PS Converter  PhysicalDomain=network_engine_domain  SubClassName=ps_input  LeftPortType=input  RightPortType=output  PseudoPeriodic=off  Frequencies=[]  NoiseDistribution=none  NoiseParameters=[]  Unit=1  AffineConversion=off  FilteringAndDerivatives=provide  SimscapeFilterOrder=1  InputFilterTimeConstant=0.001  UdotUserProvided=0
  Sine Wave : Sin  Amplitude=200  Frequency=1000  Phase=4*pi/3  SampleTime=0
  Solver Configuration : nesl_utility/Solver Configuration  PhysicalDomain=network_engine_domain  SubClassName=solver  LeftPortType=input  RightPortType=generic  Tones=[]  Harmonics=[]  SimulateNoise=off  Profile=off  UseLocalSampling=off  EnableSwitchedLinearOptims=on  FrequencyDomain=off  UseCCode=off  RelTol=0.001  AbsTol=1e-06  MinStep=1e-09  ToWorkspace=off  RevertToSquareIcSolve=off  NumHomotopyIterations=100  PhasorMode=off  PhasorModeNumHarmonics=1  DoDC=off  ResidualTolerance=1e-09  UseLocalSolver=off  LocalSolverChoice=NE_BACKWARD_EULER_ADVANCER  LocalSolverSampleTime=0.001  DoFixedCost=off  MaxNonlinIter=3  MaxModeIter=2  ComputeImpulses=off  ImpulseIterations=2  LinearAlgebra=auto  EquationFormulation=NE_TIME_EF  DelaysMemoryBudget=1024  AutomaticFiltering=on  FilteringTimeConstant=0.001  PartitionStorageMethod=AS_NEEDED  PartitionMemoryBudget=1024  PartitionMethod=ROBUST
  Voltage Sensor : fl_lib/Electrical/Electrical Sensors/Voltage Sensor
  Simulated Voltage Engine : PMIOPort  Side=Right
  Voltage engine + : PMIOPort  Port=2  Side=Right
  Voltage engine - : PMIOPort  Port=3  Side=Right
  wires:
  Sine Wave/1 -> Simulink-PS Converter/1
  connections:
  Controlled Voltage Source/RConn1 -- Simulink-PS Converter/RConn1
  Simulated Voltage Engine/RConn1 -- Voltage Sensor/RConn1
  Resistor/RConn1 -- Voltage Sensor/LConn1 -- Voltage engine +/RConn1 -- Controlled Voltage Source/LConn1
  Electrical Reference/LConn1 -- Solver Configuration/RConn1 -- Controlled Voltage Source/RConn2 -- Resistor/LConn1 -- Voltage engine -/RConn1 -- Voltage Sensor/RConn2
